simulink model "sistema_lineal_delay"  (R2018a)
settings: Solver=VariableStepAuto  StartTime=0.0  StopTime=4  RelTol=1e-3
InitFcn:
  | ini
values from neighbouring files (symbols this model uses):
  K = 1    [ini.m]
  t1 = 0.1    [ini.m]
  t2 = 0.2    [ini.m]
  wn = 3    [ini.m]
libraries: simulink x1
settings Model: Creator=cmparedes  LastModifiedBy=MarioAndres

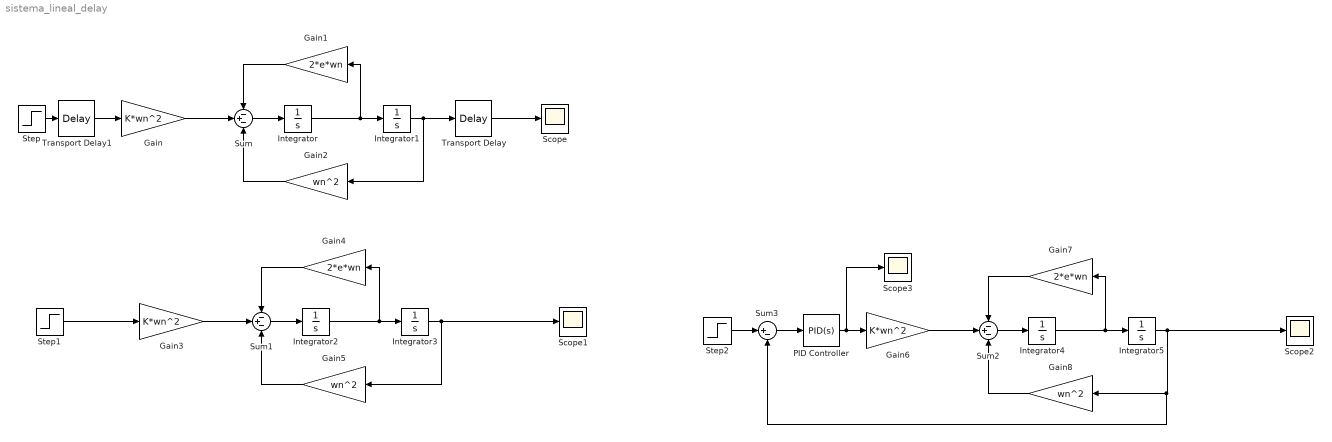
== system sistema_lineal_delay ==
  Gain : Gain  Gain=K*wn^2
  Gain1 : Gain  Gain=2*e*wn
  Gain2 : Gain  Gain=wn^2
  Gain3 : Gain  Gain=K*wn^2
  Gain4 : Gain  Gain=2*e*wn
  Gain5 : Gain  Gain=wn^2
  Gain6 : Gain  Gain=K*wn^2
  Gain7 : Gain  Gain=2*e*wn
  Gain8 : Gain  Gain=wn^2
  Integrator{,1..5} (6 alike) : Integrator
  PID Controller : simulink/Continuous/PID Controller  Controller=PID  TimeDomain=Continuous-time  SampleTime=-1  IntegratorMethod=Forward Euler  FilterMethod=Forward Euler  Form=Parallel  UseFilter=on  ControllerParametersSource=internal  P=8.6893519922945  I=14.2378395752992  D=1.24985388361572  N=71.2965664078129  InitialConditionSource=internal  InitialConditionForIntegrator=0  InitialConditionForFilter=0  ExternalReset=none  LimitOutput=off  UpperSaturationLimit=inf  LowerSaturationLimit=-inf  LinearizeAsGain=on  AntiWindupMode=none  Kb=1  TrackingMode=off  Kt=1  PParamMin=[]  PParamMax=[]  IParamMin=[]  IParamMax=[]  DParamMin=[]  DParamMax=[]  NParamMin=[]  NParamMax=[]  KbParamMin=[]  KbParamMax=[]  KtParamMin=[]  KtParamMax=[]  POutMin=[]  POutMax=[]  IOutMin=[]  IOutMax=[]  DOutMin=[]  DOutMax=[]  NOutMin=[]  NOutMax=[]  KbOutMin=[]  KbOutMax=[]  KtOutMin=[]  KtOutMax=[]  IntegratorOutMin=[]  IntegratorOutMax=[]  FilterOutMin=[]  FilterOutMax=[]  SumOutMin=[]  SumOutMax=[]  SumI1OutMin=[]  SumI1OutMax=[]  SumI2OutMin=[]  SumI2OutMax=[]  SumI3OutMin=[]  SumI3OutMax=[]  SumDOutMin=[]  SumDOutMax=[]  SaturationOutMin=[]  SaturationOutMax=[]  IntegratorContinuousStateAttributes=''  IntegratorStateMustResolveToSignalObject=off  IntegratorRTWStateStorageClass=Auto  FilterContinuousStateAttributes=''  FilterStateMustResolveToSignalObject=off  FilterRTWStateStorageClass=Auto  DifferentiatorICPrevScaledInput=0  DifferentiatorOutMin=[]  DifferentiatorOutMax=[]  FilterDiffOutCoefMin=[]  FilterDiffOutCoefMax=[]  SumDenOutMin=[]  SumDenOutMax=[]  SumNumOutMin=[]  SumNumOutMax=[]  ReciprocalOutMin=[]  ReciprocalOutMax=[]  DivideOutMin=[]  DivideOutMax=[]  TunerSelectOption=Transfer Function Based (PID Tuner App)
  Scope{,1..3} (4 alike) : Scope
  Step : Step  Time=0  SampleTime=0
  Step1 : Step  Time=0  SampleTime=0
  Step2 : Step  Time=0  SampleTime=0
  Sum : Sum  Inputs=-+-
  Sum1 : Sum  Inputs=-+-
  Sum2 : Sum  Inputs=-+-
  Sum3 : Sum  Inputs=|+-
  Transport Delay : TransportDelay  DelayTime=t2
  Transport Delay1 : TransportDelay  DelayTime=t1
  wires:
  Gain/1 -> Sum/2
  Sum/1 -> Integrator/1
  Gain1/1 -> Sum/1
  Integrator/1 -> Integrator1/1, Gain1/1
  Gain2/1 -> Sum/3
  Integrator1/1 -> Transport Delay/1, Gain2/1
  Transport Delay/1 -> Scope/1
  Step/1 -> Transport Delay1/1
  Transport Delay1/1 -> Gain/1
  Step1/1 -> Gain3/1
  Integrator3/1 -> Scope1/1, Gain5/1
  Sum1/1 -> Integrator2/1
  Gain4/1 -> Sum1/1
  Integrator2/1 -> Integrator3/1, Gain4/1
  Gain5/1 -> Sum1/3
  Gain3/1 -> Sum1/2
  Gain7/1 -> Sum2/1
  Sum2/1 -> Integrator4/1
  Integrator4/1 -> Integrator5/1, Gain7/1
  Gain8/1 -> Sum2/3
  Integrator5/1 -> Scope2/1, Sum3/2, Gain8/1
  Gain6/1 -> Sum2/2
  Step2/1 -> Sum3/1
  Sum3/1 -> PID Controller/1
  PID Controller/1 -> Scope3/1, Gain6/1
